simulink library "csc_sc_wsim_stored_command_lib"  (R2014b)
settings: Solver=ode45  StartTime=0.0  StopTime=10.0  RelTol=1e-3
values from neighbouring files (symbols this model uses):
  fsw_dt = 0.02    [csc_sc_wsim_stored_command_test.m]
  sc_empty_cmd_queue = zeros(sc_queue_depth, sc_tbl_cmd_size,'uint8')    [csc_sc_wsim_stored_command_prep.m]
  sc_num_rts = length(sc_rts_list)    [csc_rtc_rts_collection_generate.m]    (also in csc_sc_wsim_stored_command_prep.m)
  sc_queue_depth = sc_num_rts + 2    [csc_sc_wsim_stored_command_prep.m]
undefined symbols (not defined in the file or in its folder): csc_sc_dt, sc_empty_cmd_row, sc_tbl_cmd_data
libraries: simulink x8, util_common_lib x3, util_info_lib x1, csc_rtc_rts_collection_lib x1
settings Model: Creator=mstewart  LastModifiedBy=mstewart

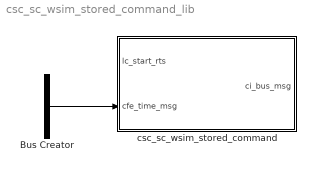
== system csc_sc_wsim_stored_command_lib ==
  Bus Creator : BusCreator  Inputs=2  OutDataTypeStr=Bus: sch_bus_msg  NonVirtualBus=on
  csc_sc_wsim_stored_command : Subsystem  TreatAsAtomicUnit=on  SystemSampleTime=csc_sc_dt
  wires:
  ? -> Bus Creator/1  "met_mseconds"
  ? -> Bus Creator/2  "met_seconds"
  Bus Creator/1 -> csc_sc_wsim_stored_command/2(cfe_time_msg)

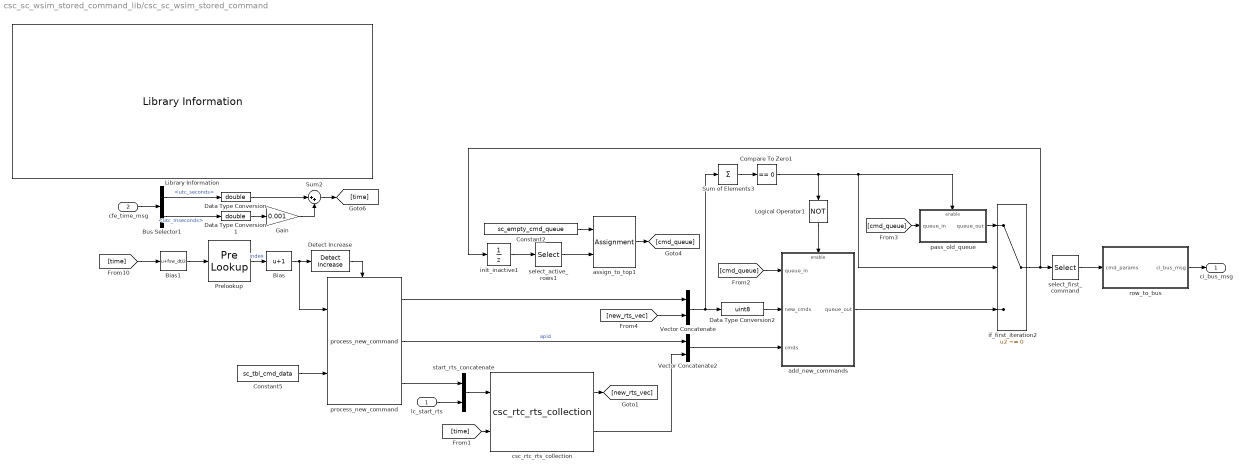
== system csc_sc_wsim_stored_command_lib/csc_sc_wsim_stored_command ==
  lc_start_rts : Inport
  cfe_time_msg : Inport  Port=2  OutDataTypeStr=Bus: cfe_time_msg
  Bias : Bias  Bias=1  SaturateOnIntegerOverflow=on
  Bias1 : Bias  Bias=fsw_dt/2  SaturateOnIntegerOverflow=on
  Bus Selector1 : BusSelector  OutputSignals=utc_seconds,utc_mseconds
  Compare To Zero1 : simulink/Logic and Bit Operations/Compare To Zero  relop===  OutDataTypeStr=boolean
  Constant2 : Constant  Value=sc_empty_cmd_queue  OutDataTypeStr=uint8
  Constant5 : Constant  Value=sc_tbl_cmd_data  OutDataTypeStr=uint8
  Data Type Conversion : DataTypeConversion  OutDataTypeStr=double
  Data Type Conversion1 : DataTypeConversion  OutDataTypeStr=double
  Data Type Conversion2 : DataTypeConversion  OutDataTypeStr=uint8
  Detect Increase : simulink/Logic and Bit Operations/Detect Increase  vinit=1  InputProcessing=Inherited  OutDataTypeStr=boolean
  Gain : Gain  Gain=0.001
  Library Information : util_info_lib/Library Information  owner='escrane'
  Logical Operator1 : Logic  Operator=NOT  AllPortsSameDT=off  OutDataTypeStr=boolean
  Prelookup : PreLookup  BreakpointsData=sc_tbl_cmd_time  BeginIndexSearchUsingPreviousIndexResult=on  OutputOnlyTheIndex=on  UseLastBreakpoint=on
  Sum of Elements3 : Sum  Inputs=+  CollapseDim=2
  Sum2 : Sum  Inputs=|++
  Vector Concatenate : Concatenate
  Vector Concatenate2 : Concatenate  Mode=Multidimensional array
  add_new_commands : Subsystem  TreatAsAtomicUnit=on
  assign_to_top1 : Assignment  NumberOfDimensions=2  IndexOptions=Index vector (dialog),Assign all  Indices=1:sc_queue_depth-1,1  OutputSizes=1,1
  csc_rtc_rts_collection : csc_rtc_rts_collection_lib/csc_rtc_rts_collection  SystemSampleTime=-1
  if_first_iteration2 : Switch  Criteria=u2 ~= 0
  init_inactive1 : UnitDelay  InitialCondition=sc_empty_cmd_queue  SampleTime=-1
  pass_old_queue : Subsystem  TreatAsAtomicUnit=on
  process_new_command : util_common_lib/process_new_command  SystemSampleTime=-1
  row_to_bus : Subsystem  TreatAsAtomicUnit=on
  select_active_rows1 : Selector  NumberOfDimensions=2  InputPortWidth=3  IndexOptions=Index vector (dialog),Select all  Indices=2:sc_queue_depth,2:sc_queue_depth  OutputSizes=1,1
  select_first_command : Selector  NumberOfDimensions=2  InputPortWidth=3  IndexOptions=Index vector (dialog),Select all  Indices=1,1  OutputSizes=1,1
  start_rts_concatenate : Concatenate
  ci_bus_msg : Outport  OutDataTypeStr=Bus: ci_cmd_msg
  wires:
  lc_start_rts/1 -> start_rts_concatenate/2
  start_rts_concatenate/1 -> csc_rtc_rts_collection/1
  process_new_command/3 -> start_rts_concatenate/1
  Data Type Conversion2/1 -> add_new_commands/2(new_cmds)
  add_new_commands/1(queue_out) -> if_first_iteration2/3
  pass_old_queue/1(queue_out) -> if_first_iteration2/1
  Logical Operator1/1 -> add_new_commands/Enable
  Compare To Zero1/1 -> Logical Operator1/1, pass_old_queue/Enable, if_first_iteration2/2
  [cmd_queue] -> pass_old_queue/1(queue_in)
  [cmd_queue] -> add_new_commands/1(queue_in)
  assign_to_top1/1 -> [cmd_queue]
  if_first_iteration2/1 -> init_inactive1/1, select_first_command/1
  Sum of Elements3/1 -> Compare To Zero1/1
  select_first_command/1 -> row_to_bus/1(cmd_params)
  Constant2/1 -> assign_to_top1/1
  select_active_rows1/1 -> assign_to_top1/2
  init_inactive1/1 -> select_active_rows1/1
  Vector Concatenate/1 -> Sum of Elements3/1, Data Type Conversion2/1
  process_new_command/1 -> Vector Concatenate/1
  Bias/1 -> process_new_command/1, Detect Increase/1
  Prelookup/1 -> Bias/1  "index"
  Constant5/1 -> process_new_command/2
  Detect Increase/1 -> process_new_command/Enable
  cfe_time_msg/1 -> Bus Selector1/1
  Bus Selector1/2 -> Data Type Conversion1/1  "<utc_mseconds>"
  Data Type Conversion/1 -> Sum2/1
  Data Type Conversion1/1 -> Gain/1
  Gain/1 -> Sum2/2
  Bus Selector1/1 -> Data Type Conversion/1  "<utc_seconds>"
  Sum2/1 -> [time]
  [time] -> Bias1/1
  row_to_bus/1(ci_bus_msg) -> ci_bus_msg/1
  Bias1/1 -> Prelookup/1
  [time] -> csc_rtc_rts_collection/2
  process_new_command/2 -> Vector Concatenate2/1  "apid"
  csc_rtc_rts_collection/2 -> Vector Concatenate2/2
  csc_rtc_rts_collection/1 -> [new_rts_vec]
  [new_rts_vec] -> Vector Concatenate/2
  Vector Concatenate2/1 -> add_new_commands/3(cmds)

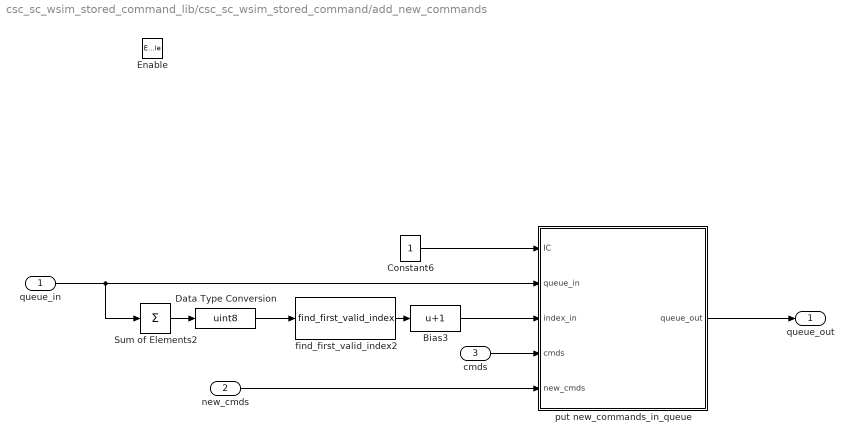
== system csc_sc_wsim_stored_command_lib/csc_sc_wsim_stored_command/add_new_commands ==
  queue_in : Inport
  new_cmds : Inport  Port=2
  cmds : Inport  Port=3
  Enable : EnablePort
  Bias3 : Bias  Bias=1  SaturateOnIntegerOverflow=on
  Constant6 : Constant  OutDataTypeStr=uint8
  Data Type Conversion : DataTypeConversion  OutDataTypeStr=uint8
  Sum of Elements2 : Sum  Inputs=+  CollapseMode=Specified dimension  CollapseDim=2  AccumDataTypeStr=uint8
  find_first_valid_index2 : util_common_lib/find_first_valid_index  vector_length=sc_queue_depth
  put new_commands_in_queue : Subsystem  TreatAsAtomicUnit=on
  queue_out : Outport
  wires:
  Data Type Conversion/1 -> find_first_valid_index2/1
  cmds/1 -> put new_commands_in_queue/4(cmds)
  new_cmds/1 -> put new_commands_in_queue/5(new_cmds)
  put new_commands_in_queue/1(queue_out) -> queue_out/1
  Constant6/1 -> put new_commands_in_queue/1(IC)
  Bias3/1 -> put new_commands_in_queue/3(index_in)
  find_first_valid_index2/1 -> Bias3/1
  Sum of Elements2/1 -> Data Type Conversion/1
  queue_in/1 -> put new_commands_in_queue/2(queue_in), Sum of Elements2/1

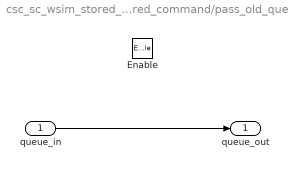
== system csc_sc_wsim_stored_command_lib/csc_sc_wsim_stored_command/pass_old_queue ==
  queue_in : Inport
  Enable : EnablePort
  queue_out : Outport
  wires:
  queue_in/1 -> queue_out/1

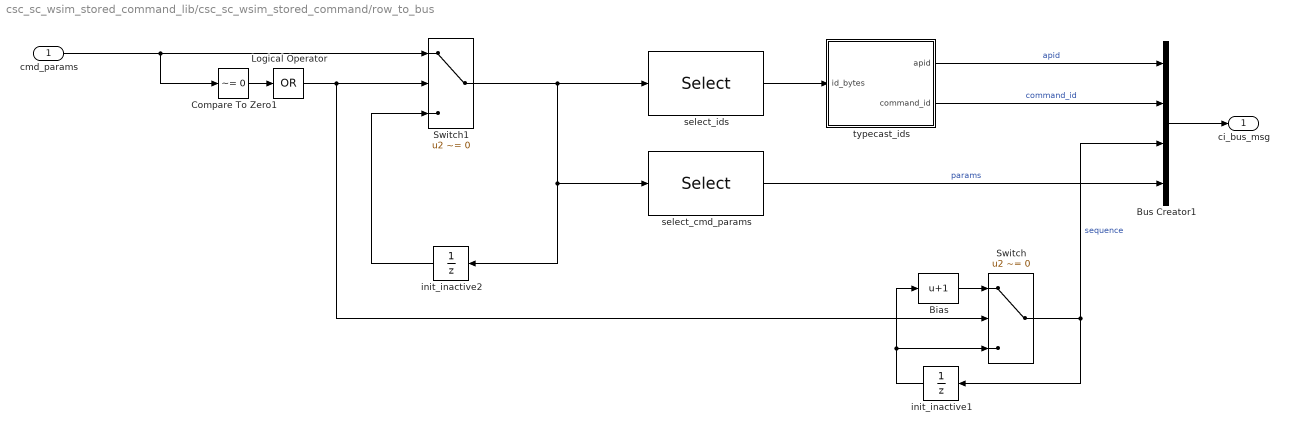
== system csc_sc_wsim_stored_command_lib/csc_sc_wsim_stored_command/row_to_bus ==
  cmd_params : Inport
  Bias : Bias  Bias=1  SaturateOnIntegerOverflow=on
  Bus Creator1 : BusCreator  OutDataTypeStr=Bus: ci_cmd_msg  NonVirtualBus=on
  Compare To Zero1 : simulink/Logic and Bit Operations/Compare To Zero  relop=~=  OutDataTypeStr=boolean
  Logical Operator : Logic  Operator=OR  Inputs=1  AllPortsSameDT=off  OutDataTypeStr=boolean
  Switch : Switch  Criteria=u2 ~= 0
  Switch1 : Switch  Criteria=u2 ~= 0
  init_inactive1 : UnitDelay  SampleTime=-1
  init_inactive2 : UnitDelay  InitialCondition=sc_empty_cmd_row  SampleTime=-1
  select_cmd_params : Selector  InputPortWidth=sc_tbl_cmd_size  Indices=sc_params_index
  select_ids : Selector  InputPortWidth=sc_tbl_cmd_size  Indices=sc_ids_index
  typecast_ids : Subsystem
  ci_bus_msg : Outport
  wires:
  Switch1/1 -> select_ids/1, init_inactive2/1, select_cmd_params/1
  init_inactive2/1 -> Switch1/3
  cmd_params/1 -> Switch1/1, Compare To Zero1/1
  Compare To Zero1/1 -> Logical Operator/1
  select_ids/1 -> typecast_ids/1(id_bytes)
  typecast_ids/2(command_id) -> Bus Creator1/2  "command_id"
  typecast_ids/1(apid) -> Bus Creator1/1  "apid"
  select_cmd_params/1 -> Bus Creator1/4  "params"
  Switch/1 -> init_inactive1/1, Bus Creator1/3  "sequence"
  Bus Creator1/1 -> ci_bus_msg/1
  Bias/1 -> Switch/1
  init_inactive1/1 -> Bias/1, Switch/3
  Logical Operator/1 -> Switch1/2, Switch/2

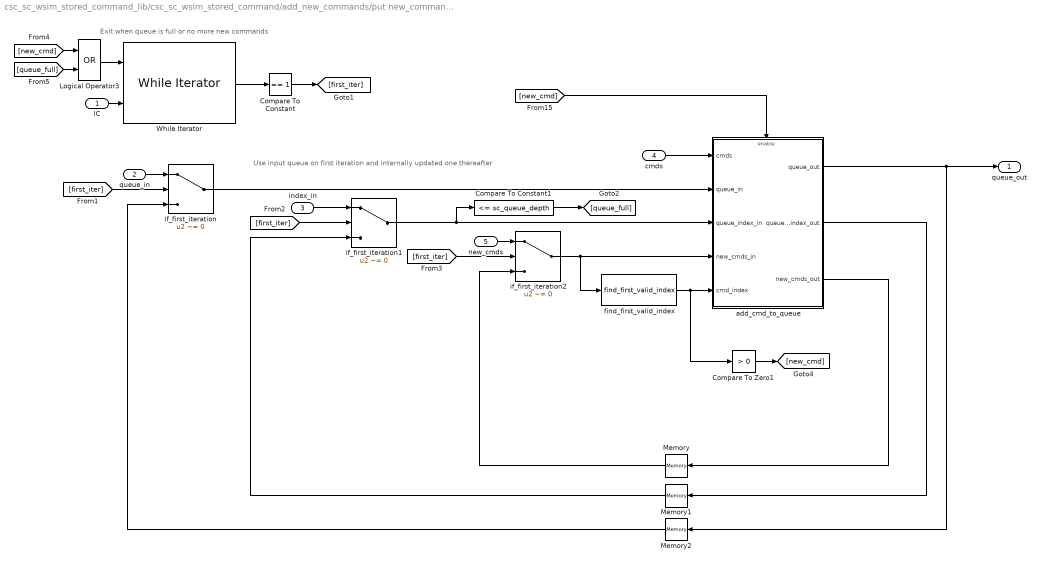
== system csc_sc_wsim_stored_command_lib/csc_sc_wsim_stored_command/add_new_commands/put new_commands_in_queue ==
  note: Exit when queue is full or no more new commands
  note: Use input queue on first iteration and internally updated one thereafter
  IC : Inport
  queue_in : Inport  Port=2
  index_in : Inport  Port=3
  cmds : Inport  Port=4
  new_cmds : Inport  Port=5
  Compare To Constant : simulink/Logic and Bit Operations/Compare To Constant  relop===  const=1  OutDataTypeStr=boolean
  Compare To Constant1 : simulink/Logic and Bit Operations/Compare To Constant  relop=<=  const=sc_queue_depth  OutDataTypeStr=boolean
  Compare To Zero1 : simulink/Logic and Bit Operations/Compare To Zero  relop=>  OutDataTypeStr=boolean
  Logical Operator3 : Logic  Operator=OR  AllPortsSameDT=off  OutDataTypeStr=boolean
  Memory : Memory  X0=uint8(zeros(sc_num_rts+1,1))  InheritSampleTime=on
  Memory1 : Memory  X0=uint32(0)  InheritSampleTime=on
  Memory2 : Memory  X0=sc_empty_cmd_queue  InheritSampleTime=on
  While Iterator : WhileIterator  MaxIters=sc_queue_depth  ShowIterationPort=on
  add_cmd_to_queue : Subsystem  TreatAsAtomicUnit=on
  find_first_valid_index : util_common_lib/find_first_valid_index  vector_length=sc_num_rts+1
  if_first_iteration : Switch  Criteria=u2 ~= 0  OutDataTypeStr=uint8
  if_first_iteration1 : Switch  Criteria=u2 ~= 0  OutDataTypeStr=uint32
  if_first_iteration2 : Switch  Criteria=u2 ~= 0  OutDataTypeStr=uint8
  queue_out : Outport
  wires:
  [queue_full] -> Logical Operator3/2
  [new_cmd] -> Logical Operator3/1
  Logical Operator3/1 -> While Iterator/1
  Compare To Constant1/1 -> [queue_full]
  Compare To Constant/1 -> [first_iter]
  Memory2/1 -> if_first_iteration/3
  Memory1/1 -> if_first_iteration1/3
  Memory/1 -> if_first_iteration2/3
  find_first_valid_index/1 -> add_cmd_to_queue/5(cmd_index), Compare To Zero1/1
  Compare To Zero1/1 -> [new_cmd]
  new_cmds/1 -> if_first_iteration2/1
  if_first_iteration2/1 -> add_cmd_to_queue/4(new_cmds_in), find_first_valid_index/1
  [first_iter] -> if_first_iteration2/2
  add_cmd_to_queue/3(new_cmds_out) -> Memory/1
  if_first_iteration1/1 -> add_cmd_to_queue/3(queue_index_in), Compare To Constant1/1
  if_first_iteration/1 -> add_cmd_to_queue/2(queue_in)
  add_cmd_to_queue/2(queue_index_out) -> Memory1/1
  index_in/1 -> if_first_iteration1/1
  [first_iter] -> if_first_iteration1/2
  add_cmd_to_queue/1(queue_out) -> Memory2/1, queue_out/1
  queue_in/1 -> if_first_iteration/1
  [first_iter] -> if_first_iteration/2
  While Iterator/1 -> Compare To Constant/1
  cmds/1 -> add_cmd_to_queue/1(cmds)
  [new_cmd] -> add_cmd_to_queue/Enable
  IC/1 -> While Iterator/2

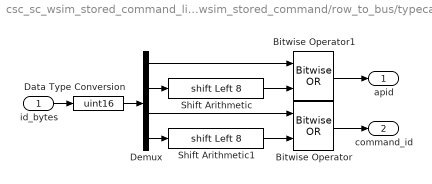
== system csc_sc_wsim_stored_command_lib/csc_sc_wsim_stored_command/row_to_bus/typecast_ids ==
  id_bytes : Inport
  Bitwise Operator : simulink/Logic and Bit Operations/Bitwise Operator  logicop=OR  UseBitMask=off  NumInputPorts=2  BitMask=bin2dec('11011001')  BitMaskRealWorld=Stored Integer
  Bitwise Operator1 : simulink/Logic and Bit Operations/Bitwise Operator  logicop=OR  UseBitMask=off  NumInputPorts=2  BitMask=bin2dec('11011001')  BitMaskRealWorld=Stored Integer
  Data Type Conversion : DataTypeConversion  OutDataTypeStr=uint16
  Demux : Demux
  Shift Arithmetic : ArithShift  BitShiftNumber=8  BitShiftDirection=Left
  Shift Arithmetic1 : ArithShift  BitShiftNumber=8  BitShiftDirection=Left
  apid : Outport
  command_id : Outport  Port=2
  wires:
  id_bytes/1 -> Data Type Conversion/1
  Data Type Conversion/1 -> Demux/1
  Demux/2 -> Shift Arithmetic/1
  Demux/4 -> Shift Arithmetic1/1
  Shift Arithmetic1/1 -> Bitwise Operator/2
  Demux/3 -> Bitwise Operator/1
  Shift Arithmetic/1 -> Bitwise Operator1/2
  Demux/1 -> Bitwise Operator1/1
  Bitwise Operator/1 -> command_id/1
  Bitwise Operator1/1 -> apid/1

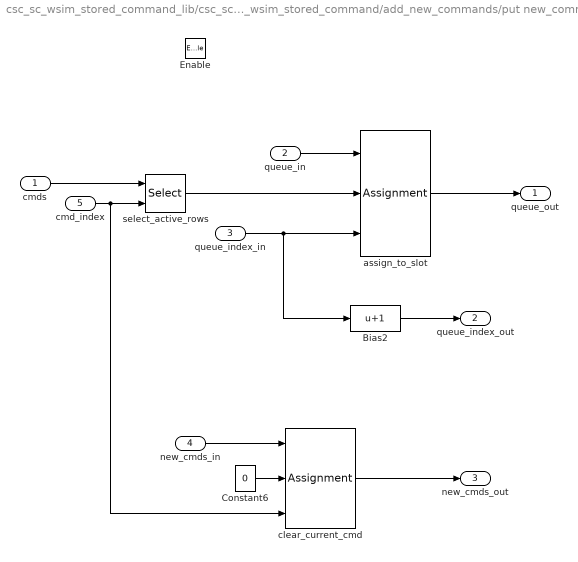
== system csc_sc_wsim_stored_command_lib/csc_sc_wsim_stored_command/add_new_commands/put new_commands_in_queue/add_cmd_to_queue ==
  cmds : Inport
  queue_in : Inport  Port=2
  queue_index_in : Inport  Port=3
  new_cmds_in : Inport  Port=4
  cmd_index : Inport  Port=5
  Enable : EnablePort
  Bias2 : Bias  Bias=1  SaturateOnIntegerOverflow=on
  Constant6 : Constant  Value=0  OutDataTypeStr=uint8
  assign_to_slot : Assignment  NumberOfDimensions=2  IndexOptions=Index vector (port),Assign all  Indices=1,1  OutputSizes=1,1
  clear_current_cmd : Assignment  IndexOptions=Index vector (port)
  select_active_rows : Selector  NumberOfDimensions=2  InputPortWidth=3  IndexOptions=Index vector (port),Select all  Indices=[1 3],2:sc_queue_depth  OutputSizes=1,1
  queue_out : Outport
  queue_index_out : Outport  Port=2
  new_cmds_out : Outport  Port=3
  wires:
  Constant6/1 -> clear_current_cmd/2
  clear_current_cmd/1 -> new_cmds_out/1
  new_cmds_in/1 -> clear_current_cmd/1
  cmd_index/1 -> select_active_rows/2, clear_current_cmd/3
  select_active_rows/1 -> assign_to_slot/2
  Bias2/1 -> queue_index_out/1
  assign_to_slot/1 -> queue_out/1
  cmds/1 -> select_active_rows/1
  queue_index_in/1 -> assign_to_slot/3, Bias2/1
  queue_in/1 -> assign_to_slot/1
